simulink model "Receive_Ethernet_UDP_2024a"  (R2024a)
settings: Solver=FixedStepAuto  StartTime=0.0  StopTime=inf  FixedStep=0.01  RelTol=1e-3
undefined symbols (not defined in the file): f, gray
libraries: instrumentlib x4, etargetslib x1
settings Model: Creator=hyeon-yongjeong  LastModifiedBy=hyeon-yongjeong

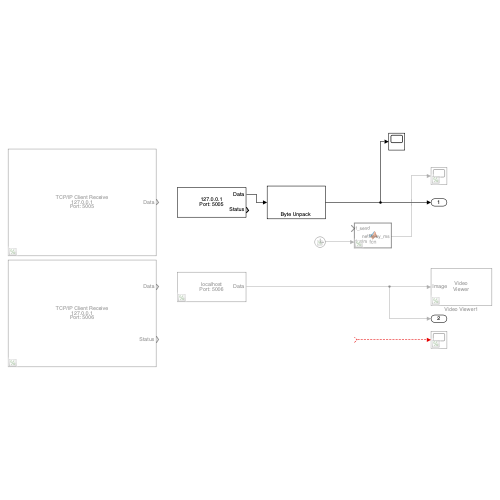
[thumbnail: Simulink's stored preview of the top-level diagram]
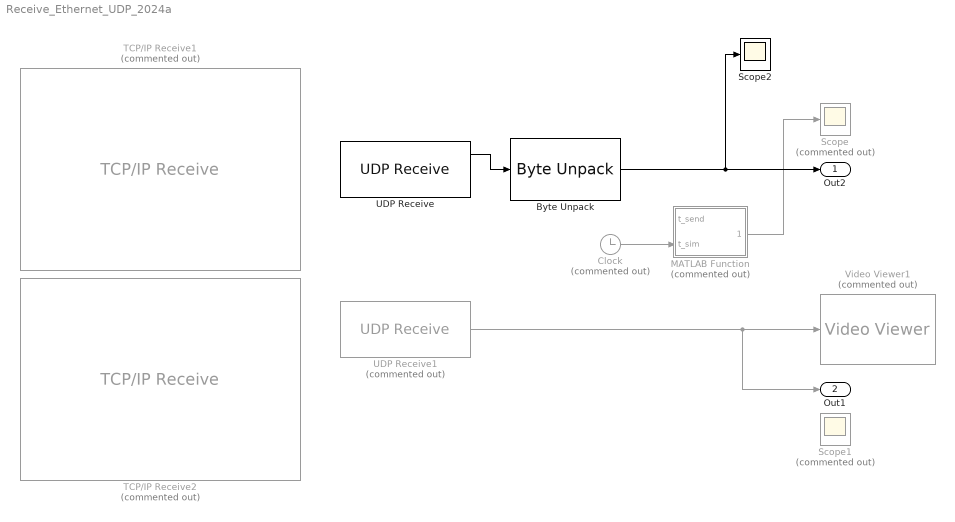
== system Receive_Ethernet_UDP_2024a ==
  Byte Unpack : etargetslib/Byte Unpack  dimensions={[9 1]}  datatypes={'double'}  byteAlign=8
      settings: LibrarySourceBlock=embeddedtargetslib/Host Communication/Byte Unpack
  Clock : Clock  Commented=on
  MATLAB Function : MATLAB Function  Commented=on  TreatAsAtomicUnit=on
  Scope : Scope  Commented=on
  Scope1 : Scope  Commented=on
  Scope2 : Scope
  TCP/IP Receive1 : instrumentlib/TCP//IP Receive  Commented=on  Host=127.0.0.1  Port=5005  DataSize=[ 7 1 ]  DataType=single  ASCIIFormatting=%f  Terminator=LF  CustomTerminator=10  ByteOrder=little-endian  EnableBlockingMode=on  Timeout=10  SampleTime=0.01  SimulateUsing=Interpreted execution
  TCP/IP Receive2 : instrumentlib/TCP//IP Receive  Commented=on  Host=127.0.0.1  Port=5006  DataSize=[240 320]  DataType=uint8  ASCIIFormatting=%f  Terminator=LF  CustomTerminator=10  ByteOrder=little-endian  EnableBlockingMode=off  Timeout=10  SampleTime=0.01  SimulateUsing=Interpreted execution
  UDP Receive : instrumentlib/UDP Receive  LocalAddress=127.0.0.1  LocalPort=5005  EnablePortSharing=off  Host=0.0.0.0  Port=5005  GetLatestData=off  DataSize=[8*9 1 ]  DataType=uint8  ASCIIFormatting=%f,  Terminator=LF  CustomTerminator=10  ByteOrder=big-endian  EnableBlockingMode=off  Timeout=10  SampleTime=0.01  SimulateUsing=Interpreted execution
  UDP Receive1 : instrumentlib/UDP Receive  Commented=on  LocalAddress=localhost  LocalPort=5006  EnablePortSharing=off  Host=localhost  Port=5006  GetLatestData=off  DataSize=[240 320]  DataType=uint8  ASCIIFormatting=%f,  Terminator=LF  CustomTerminator=10  ByteOrder=big-endian  EnableBlockingMode=on  Timeout=10  SampleTime=0.01  SimulateUsing=Interpreted execution
  Video Viewer1 : VideoViewer  Commented=on  colormapValue=gray(256)  FigPos=[951 720 636 450]
  Out2 : Outport
  Out1 : Outport  Port=2
  wires:
  UDP Receive1/1 -> Out1/1, Video Viewer1/1
  ? -> Scope1/1
  Clock/1 -> MATLAB Function/2(t_sim)
  MATLAB Function/1(netDelay_ms) -> Scope/1
  Byte Unpack/1 -> Scope2/1, Out2/1
  UDP Receive/1 -> Byte Unpack/1

== matlab function Receive_Ethernet_UDP_2024a/MATLAB Function ==
  data: t_send input; netDelay_ms output; t_sim input
function netDelay_ms  = fcn(t_send, t_sim)
  netDelay_ms = (t_sim - t_send) * 1e3;
end
